simulink model "mancal_v2_corsi"  (R2013a)
settings: Solver=ode45  StartTime=0.0  StopTime=3  RelTol=1e-5
values from neighbouring files (symbols this model uses):
  dA = [1.435e2 3.335e-2]    [parametriza.m]    (also in parametrizaMancal.m)
  E = 3e9    (= 3000000000)    [parametriza.m]    (also in parametrizaMancal.m)
  gb = 0.4e-3    (= 0.0004)    [main.m]    (also in parametriza.m = 0.0003; parametrizaMancal.m)
  gi = 0.6e-3    (= 0.0006)    [main.m]    (also in parametriza.m = 0.0007; parametrizaMancal.m)
  Hb = 8e-3    (= 0.008)    [parametriza.m]    (also in parametrizaMancal.m)
  Kb = 46.53E3    (= 46530)    [main.m]    (also in parametriza.m = 58; parametrizaMancal.m = E*Hb*Ab/Lb)
  Ke = [3.8e-9 2.86e-3]    [parametrizaMancal.m]
  Km = 540e3    (= 540000)    [parametrizaMancal.m]
  L = [-57.6135 0.0908]    [main.m]    (also in parametriza.m = tf(Kb,[L2 R]); parametrizaMancal.m)
  Lb = 5.3e-3    (= 0.0053)    [parametriza.m]    (also in parametrizaMancal.m)
  m = 4.7e-5*7.86e3    (= 0.36942)    [main.m]    (also in parametriza.m = 0.375; parametrizaMancal.m)
  N = 300    [main.m]    (also in parametriza.m; parametrizaMancal.m)
  R = 4    [main.m]    (also in parametriza.m = 6.3; parametrizaMancal.m)
  Vmax = 30    [parametriza.m]    (also in parametrizaMancal.m)
undefined symbols (not defined in the file or in its folder): C
libraries: simulink x1, dspmathops x1
settings Model: SimulationMode=accelerator  Creator=leo  LastModifiedBy=rafa
settings DataIOCC: SignalLoggingSaveFormat=ModelDataLogs
settings OptimizationCC: AccelVerboseBuild=on
settings DebuggingCC: SolverPrmCheckMsg=none  MultiTaskDSMMsg=warning  MultiTaskCondExecSysMsg=none  StrictBusMsg=None
settings ModelReferenceCC: UpdateModelReferenceTargets=IfOutOfDate
settings SFSimCC: SFSimEcho=off
settings RTWCC: IncludeERTFirstTime=on

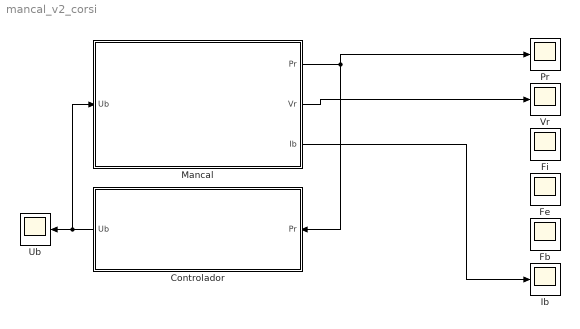
== system mancal_v2_corsi ==
  Controlador : Subsystem
  Fb : Scope
      settings: YMin=-200000  YMax=200000  SaveName=ScopeData6
  Fe : Scope
      settings: YMin=-500  YMax=25  SaveName=ScopeData2
  Fi : Scope
      settings: YMin=0  YMax=450  SaveName=ScopeData3
  Ib : Scope
      settings: YMin=-4  YMax=4  SaveName=ScopeData5
  Mancal : Subsystem
  Pr : Scope
      settings: TimeRange=3  YMin=-0.00045  YMax=0.00045
  Ub : Scope
      settings: TimeRange=0.1  YMin=0  YMax=10  SaveName=ScopeData10
  Vr : Scope
      settings: YMin=-45  YMax=45
  wires:
  Mancal/1(Pr) -> Pr/1, Controlador/1(Pr)
  Mancal/2(Vr) -> Vr/1
  ? -> Fe/1
  ? -> Fi/1
  Mancal/3(Ib) -> Ib/1
  ? -> Fb/1
  Controlador/1(Ub) -> Ub/1, Mancal/1(Ub)

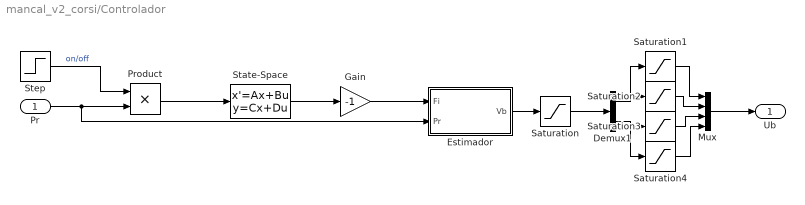
== system mancal_v2_corsi/Controlador ==
  Pr : Inport
  Demux1 : Demux  Outputs=2
  Estimador : Subsystem
  Gain : Gain  Gain=-1
  Mux : Mux
  Product : Product
  Saturation : Saturate  UpperLimit=Vmax  LowerLimit=-Vmax
  Saturation1 : Saturate  UpperLimit=Inf  LowerLimit=0
  Saturation2 : Saturate  UpperLimit=0  LowerLimit=-Inf
  Saturation3 : Saturate  UpperLimit=Inf  LowerLimit=0
  Saturation4 : Saturate  UpperLimit=0  LowerLimit=-Inf
  State-Space : StateSpace  A=ss([C 1; 1 C]).A  B=ss([C 1; 1 C]).B  C=ss([C 1; 1 C]).C  D=ss([C 1; 1 C]).D
  Step : Step  SampleTime=0
  Ub : Outport
  wires:
  Mux/1 -> Ub/1
  Saturation/1 -> Demux1/1
  Saturation4/1 -> Mux/4
  Saturation3/1 -> Mux/3
  Saturation2/1 -> Mux/2
  Saturation1/1 -> Mux/1
  Demux1/2 -> Saturation3/1, Saturation4/1
  Demux1/1 -> Saturation2/1, Saturation1/1
  Gain/1 -> Estimador/1(Fi)
  Estimador/1(Vb) -> Saturation/1
  State-Space/1 -> Gain/1
  Product/1 -> State-Space/1
  Pr/1 -> Product/2, Estimador/2(Pr)
  Step/1 -> Product/1  "on/off"

== system mancal_v2_corsi/Mancal ==
  Ub : Inport
  Batente : Subsystem
  Enrolamentos : Subsystem
  Imas : Subsystem
  Rotor : Subsystem
  Sum : Sum  Inputs=+++
  Pr : Outport
  Vr : Outport  Port=2
  Ib : Outport  Port=3
  wires:
  Sum/1 -> Rotor/1(Fr)  "F"
  Ub/1 -> Enrolamentos/1(Ub)
  Enrolamentos/1(Fe) -> Sum/3
  ? -> Ib/1
  Batente/1(Fb) -> Sum/1
  Rotor/1(Pr) -> Pr/1, Batente/1(Pr), Imas/1(Pr), Enrolamentos/2(Pr)
  Rotor/2(Vr) -> Batente/2(Vr), Vr/1
  Imas/1(Fi) -> Sum/2

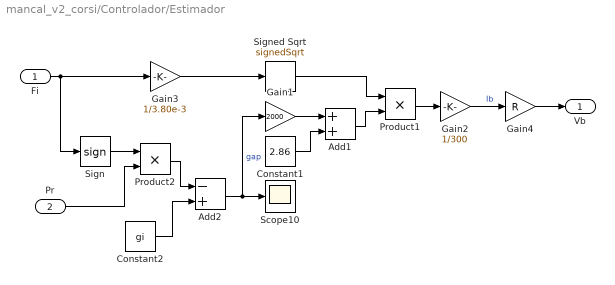
== system mancal_v2_corsi/Controlador/Estimador ==
  Fi : Inport
  Pr : Inport  Port=2
  Add1 : Sum
  Add2 : Sum  Inputs=-+
  Constant1 : Constant  Value=2.86
  Constant2 : Constant  Value=gi
  Gain1 : Gain  Gain=2000
  Gain2 : Gain  Gain=1/300
  Gain3 : Gain  Gain=1/3.80e-3
  Gain4 : Gain  Gain=R
  Product1 : Product
  Product2 : Product
  Scope10 : Scope
      settings: TimeRange=2.85171102661597  YMin=0.00015  YMax=0.0006  SaveName=ScopeData11
  Sign : Signum
  Signed Sqrt : Sqrt  Operator=signedSqrt  SaturateOnIntegerOverflow=on
  Vb : Outport
  wires:
  Constant2/1 -> Add2/2
  Product2/1 -> Add2/1
  Pr/1 -> Product2/2
  Sign/1 -> Product2/1
  Gain4/1 -> Vb/1
  Product1/1 -> Gain2/1
  Add2/1 -> Scope10/1, Gain1/1  "gap"
  Constant1/1 -> Add1/2
  Signed Sqrt/1 -> Product1/1
  Gain2/1 -> Gain4/1  "Ib"
  Gain3/1 -> Signed Sqrt/1
  Gain1/1 -> Add1/1
  Fi/1 -> Sign/1, Gain3/1
  Add1/1 -> Product1/2

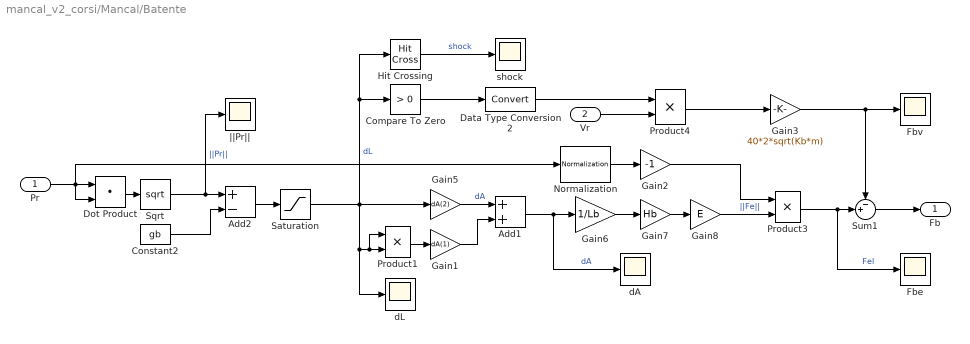
== system mancal_v2_corsi/Mancal/Batente ==
  Pr : Inport
  Vr : Inport  Port=2
  Add1 : Sum
  Add2 : Sum  Inputs=+-
  Compare To Zero : simulink/Logic and Bit Operations/Compare To Zero  relop=>  OutDataTypeStr=boolean
  Constant2 : Constant  Value=gb
  Data Type Conversion2 : DataTypeConversion
  Dot Product : DotProduct  InputSameDT=on  OutDataTypeStr=Inherit: Inherit via internal rule
  Fbe : Scope
      settings: TimeRange=0.0002829354553492485  YMin=-100000  YMax=100000  SaveName=ScopeData15
  Fbv : Scope
      settings: TimeRange=0.1  YMin=-225000  YMax=225000  SaveName=ScopeData8
  Gain1 : Gain  Gain=dA(1)
  Gain2 : Gain  Gain=-1
  Gain3 : Gain  Gain=40*2*sqrt(Kb*m)
  Gain5 : Gain  Gain=dA(2)
  Gain6 : Gain  Gain=1/Lb
  Gain7 : Gain  Gain=Hb
  Gain8 : Gain  Gain=E
  Hit Crossing : HitCross  HitCrossingDirection=rising
  Normalization : dspmathops/Normalization  NormType=2-norm  Bias=1e-10  NormOver=Each column  ColComp=on  Dimension=1  outputDataTypeStr=Inherit: Same as product output  outputLastDataTypeStr=Inherit: Same as product output  outputMin=[]  outputMax=[]  accumDataTypeStr=Inherit: Same as product output  accumLastDataTypeStr=Inherit: Same as product output  roundingMode=Floor  overflowMode=off
  Product1 : Product
  Product3 : Product
  Product4 : Product
  Saturation : Saturate  UpperLimit=Inf  LowerLimit=0
  Sqrt : Sqrt  SaturateOnIntegerOverflow=on
  Sum1 : Sum  Inputs=-+|
  dA : Scope
      settings: TimeRange=0.0002829354553492485  YMin=3.91545e-05  YMax=3.9158e-05  SaveName=ScopeData4
  dL : Scope
      settings: TimeRange=0.1  YMin=1.4215e-06  YMax=1.4315e-06  SaveName=ScopeData7
  shock : Scope
      settings: TimeRange=0.0002829354553492485  YMin=5.54637e-16  YMax=5.54639e-16  SaveName=ScopeData19
  ||Pr|| : Scope
      settings: TimeRange=0.0002829354553492485  YMin=-2.75  YMax=0  SaveName=ScopeData18
  Fb : Outport
  wires:
  Dot Product/1 -> Sqrt/1
  Gain8/1 -> Product3/2  "||Fe||"
  Compare To Zero/1 -> Data Type Conversion2/1
  Saturation/1 -> dL/1, Product1/1, Product1/2, Hit Crossing/1, Compare To Zero/1, Gain5/1  "dL"
  Add2/1 -> Saturation/1
  Sqrt/1 -> ||Pr||/1, Add2/1  "||Pr||"
  Constant2/1 -> Add2/2
  Gain6/1 -> Gain7/1
  Gain7/1 -> Gain8/1
  Product4/1 -> Gain3/1
  Product3/1 -> Sum1/2, Fbe/1  "Fel"
  Sum1/1 -> Fb/1
  Data Type Conversion2/1 -> Product4/1
  Product1/1 -> Gain1/1
  Gain5/1 -> Add1/1  "dA"
  Add1/1 -> dA/1, Gain6/1  "dA"
  Gain3/1 -> Fbv/1, Sum1/1
  Vr/1 -> Product4/2
  Normalization/1 -> Gain2/1
  Pr/1 -> Normalization/1, Dot Product/2, Dot Product/1
  Gain2/1 -> Product3/1
  Gain1/1 -> Add1/2
  Hit Crossing/1 -> shock/1  "shock"

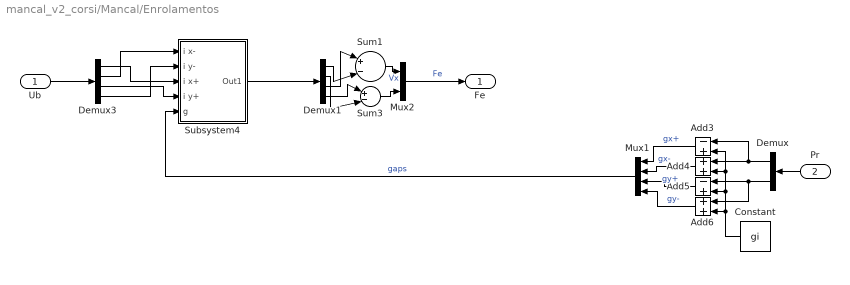
== system mancal_v2_corsi/Mancal/Enrolamentos ==
  Ub : Inport
  Pr : Inport  Port=2
  Add3 : Sum  Inputs=-+
  Add4 : Sum
  Add5 : Sum  Inputs=-+
  Add6 : Sum
  Constant : Constant  Value=gi
  Demux : Demux  Outputs=2
  Demux1 : Demux
  Demux3 : Demux
  Mux1 : Mux
  Mux2 : Mux  Inputs=2
  Subsystem4 : Subsystem
  Sum1 : Sum  Inputs=|+-|
  Sum3 : Sum  Inputs=|+-|
  Fe : Outport
  wires:
  Constant/1 -> Add5/2, Add4/2, Add3/2, Add6/2
  Mux2/1 -> Fe/1  "Fe"
  Sum3/1 -> Mux2/2
  Sum1/1 -> Mux2/1  "Vx"
  Add3/1 -> Mux1/1  "gx+"
  Add4/1 -> Mux1/2  "gx-"
  Add5/1 -> Mux1/3  "gy+"
  Add6/1 -> Mux1/4  "gy-"
  Demux/1 -> Add4/1, Add3/1
  Demux/2 -> Add5/1, Add6/1
  Pr/1 -> Demux/1
  Ub/1 -> Demux3/1
  Demux3/1 -> Subsystem4/3(i x+)
  Demux3/2 -> Subsystem4/1(i x-)
  Demux3/3 -> Subsystem4/4(i y+)
  Demux3/4 -> Subsystem4/2(i y-)
  Mux1/1 -> Subsystem4/5(g)  "gaps"
  Subsystem4/1(Out1) -> Demux1/1
  Demux1/3 -> Sum1/1
  Demux1/1 -> Sum1/2
  Demux1/4 -> Sum3/1
  Demux1/2 -> Sum3/2

== system mancal_v2_corsi/Mancal/Imas ==
  Pr : Inport
  Gain1 : Gain  Gain=Km
  Fi : Outport
  wires:
  Pr/1 -> Gain1/1
  Gain1/1 -> Fi/1  "Fm"

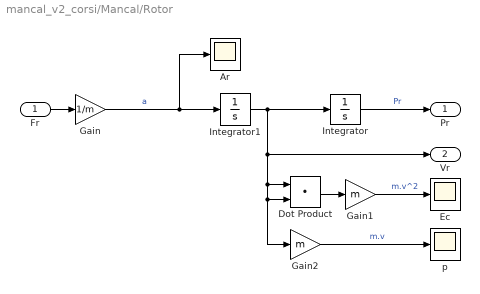
== system mancal_v2_corsi/Mancal/Rotor ==
  Fr : Inport
  Ar : Scope
      settings: TimeRange=1  YMin=-200000  YMax=200000  SaveName=ScopeData9
  Dot Product : DotProduct  InputSameDT=on  OutDataTypeStr=Inherit: Inherit via internal rule
  Ec : Scope
      settings: TimeRange=0.25  YMin=0  YMax=0.09  SaveName=ScopeData16
  Gain : Gain  Gain=1/m
  Gain1 : Gain  Gain=m
  Gain2 : Gain  Gain=m
  Integrator : Integrator  InitialCondition=[.001 .002]*1e-3  UpperSaturationLimit=Inf  LowerSaturationLimit=-Inf
  Integrator1 : Integrator
  p : Scope
      settings: TimeRange=1  YMin=-200000  YMax=200000  SaveName=ScopeData17
  Pr : Outport
  Vr : Outport  Port=2
  wires:
  Fr/1 -> Gain/1
  Integrator/1 -> Pr/1  "Pr"
  Gain/1 -> Ar/1, Integrator1/1  "a"
  Dot Product/1 -> Gain1/1
  Integrator1/1 -> Dot Product/1, Gain2/1, Dot Product/2, Vr/1, Integrator/1
  Gain2/1 -> p/1  "m.v"
  Gain1/1 -> Ec/1  "m.v^2"

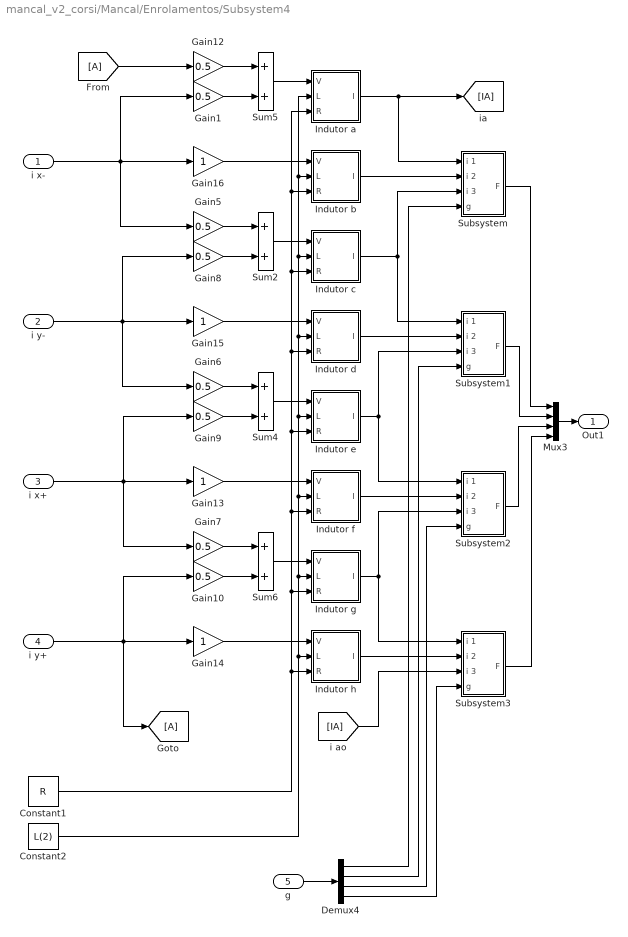
== system mancal_v2_corsi/Mancal/Enrolamentos/Subsystem4 ==
  i x- : Inport
  i y- : Inport  Port=2
  i x+ : Inport  Port=3
  i y+ : Inport  Port=4
  g : Inport  Port=5
  Constant1 : Constant  Value=R
  Constant2 : Constant  Value=L(2)
  Demux4 : Demux
  Gain{1,5..10,12} (8 alike) : Gain  Gain=0.5
  Gain{13..16} (4 alike) : Gain
  Indutor a : Subsystem
  Indutor b : Subsystem
  Indutor c : Subsystem
  Indutor d : Subsystem
  Indutor e : Subsystem
  Indutor f : Subsystem
  Indutor g : Subsystem
  Indutor h : Subsystem
  Mux3 : Mux
  Subsystem : Subsystem
  Subsystem1 : Subsystem
  Subsystem2 : Subsystem
  Subsystem3 : Subsystem
  Sum{2,4..6} (4 alike) : Sum
  Out1 : Outport
  wires:
  Sum6/1 -> Indutor g/1(V)
  i y+/1 -> [A], Gain10/1, Gain14/1
  [A] -> Gain12/1
  Gain13/1 -> Indutor f/1(V)
  Gain12/1 -> Sum5/1
  g/1 -> Demux4/1
  Demux4/3 -> Subsystem2/4(g)
  Indutor a/1(I) -> [IA], Subsystem/1(i 1)
  Subsystem/1(F) -> Mux3/1
  Demux4/1 -> Subsystem/4(g)
  Demux4/2 -> Subsystem1/4(g)
  Mux3/1 -> Out1/1
  Constant2/1 -> Indutor a/2(L), Indutor b/2(L), Indutor c/2(L), Indutor d/2(L), Indutor e/2(L), Indutor f/2(L), Indutor g/2(L), Indutor h/2(L)
  [IA] -> Subsystem3/3(i 3)
  Constant1/1 -> Indutor e/3(R), Indutor a/3(R), Indutor b/3(R), Indutor c/3(R), Indutor d/3(R), Indutor f/3(R), Indutor g/3(R), Indutor h/3(R)
  Demux4/4 -> Subsystem3/4(g)
  Subsystem3/1(F) -> Mux3/4
  Subsystem1/1(F) -> Mux3/2
  Indutor g/1(I) -> Subsystem2/3(i 3), Subsystem3/1(i 1)
  Indutor c/1(I) -> Subsystem/3(i 3), Subsystem1/1(i 1)
  Indutor d/1(I) -> Subsystem1/2(i 2)
  Indutor h/1(I) -> Subsystem3/2(i 2)
  Indutor e/1(I) -> Subsystem1/3(i 3), Subsystem2/1(i 1)
  Gain14/1 -> Indutor h/1(V)
  Gain15/1 -> Indutor d/1(V)
  Gain16/1 -> Indutor b/1(V)
  Indutor b/1(I) -> Subsystem/2(i 2)
  Sum5/1 -> Indutor a/1(V)
  Gain9/1 -> Sum4/2
  i x+/1 -> Gain7/1, Gain13/1, Gain9/1
  Gain10/1 -> Sum6/2
  Subsystem2/1(F) -> Mux3/3
  Indutor f/1(I) -> Subsystem2/2(i 2)
  i y-/1 -> Gain15/1, Gain8/1, Gain6/1
  Gain6/1 -> Sum4/1
  Sum4/1 -> Indutor e/1(V)
  Gain8/1 -> Sum2/2
  Gain7/1 -> Sum6/1
  Gain1/1 -> Sum5/2
  i x-/1 -> Gain1/1, Gain5/1, Gain16/1
  Sum2/1 -> Indutor c/1(V)
  Gain5/1 -> Sum2/1

== system mancal_v2_corsi/Mancal/Enrolamentos/Subsystem4/Indutor a ==
  V : Inport
  L : Inport  Port=2
  R : Inport  Port=3
  Divide2 : Product  Inputs=*/
  Integrator : Integrator
  Product : Product
  Sum1 : Sum  Inputs=|+-
  I : Outport
  wires:
  Divide2/1 -> Integrator/1
  Sum1/1 -> Divide2/1
  Integrator/1 -> Product/1, I/1
  Product/1 -> Sum1/2
  L/1 -> Divide2/2
  V/1 -> Sum1/1
  R/1 -> Product/2

== system mancal_v2_corsi/Mancal/Enrolamentos/Subsystem4/Indutor b ==
  V : Inport
  L : Inport  Port=2
  R : Inport  Port=3
  Divide2 : Product  Inputs=*/
  Integrator : Integrator
  Product : Product
  Sum1 : Sum  Inputs=|+-
  I : Outport
  wires:
  Divide2/1 -> Integrator/1
  Sum1/1 -> Divide2/1
  Integrator/1 -> Product/1, I/1
  Product/1 -> Sum1/2
  L/1 -> Divide2/2
  V/1 -> Sum1/1
  R/1 -> Product/2

== system mancal_v2_corsi/Mancal/Enrolamentos/Subsystem4/Indutor c ==
  V : Inport
  L : Inport  Port=2
  R : Inport  Port=3
  Divide2 : Product  Inputs=*/
  Integrator : Integrator
  Product : Product
  Sum1 : Sum  Inputs=|+-
  I : Outport
  wires:
  Divide2/1 -> Integrator/1
  Sum1/1 -> Divide2/1
  Integrator/1 -> Product/1, I/1
  Product/1 -> Sum1/2
  L/1 -> Divide2/2
  V/1 -> Sum1/1
  R/1 -> Product/2

== system mancal_v2_corsi/Mancal/Enrolamentos/Subsystem4/Indutor d ==
  V : Inport
  L : Inport  Port=2
  R : Inport  Port=3
  Divide2 : Product  Inputs=*/
  Integrator : Integrator
  Product : Product
  Sum1 : Sum  Inputs=|+-
  I : Outport
  wires:
  Divide2/1 -> Integrator/1
  Sum1/1 -> Divide2/1
  Integrator/1 -> Product/1, I/1
  Product/1 -> Sum1/2
  L/1 -> Divide2/2
  V/1 -> Sum1/1
  R/1 -> Product/2

== system mancal_v2_corsi/Mancal/Enrolamentos/Subsystem4/Indutor e ==
  V : Inport
  L : Inport  Port=2
  R : Inport  Port=3
  Divide2 : Product  Inputs=*/
  Integrator : Integrator
  Product : Product
  Sum1 : Sum  Inputs=|+-
  I : Outport
  wires:
  Divide2/1 -> Integrator/1
  Sum1/1 -> Divide2/1
  Integrator/1 -> Product/1, I/1
  Product/1 -> Sum1/2
  L/1 -> Divide2/2
  V/1 -> Sum1/1
  R/1 -> Product/2

== system mancal_v2_corsi/Mancal/Enrolamentos/Subsystem4/Indutor f ==
  V : Inport
  L : Inport  Port=2
  R : Inport  Port=3
  Divide2 : Product  Inputs=*/
  Integrator : Integrator
  Product : Product
  Sum1 : Sum  Inputs=|+-
  I : Outport
  wires:
  Divide2/1 -> Integrator/1
  Sum1/1 -> Divide2/1
  Integrator/1 -> Product/1, I/1
  Product/1 -> Sum1/2
  L/1 -> Divide2/2
  V/1 -> Sum1/1
  R/1 -> Product/2

== system mancal_v2_corsi/Mancal/Enrolamentos/Subsystem4/Indutor g ==
  V : Inport
  L : Inport  Port=2
  R : Inport  Port=3
  Divide2 : Product  Inputs=*/
  Integrator : Integrator
  Product : Product
  Sum1 : Sum  Inputs=|+-
  I : Outport
  wires:
  Divide2/1 -> Integrator/1
  Sum1/1 -> Divide2/1
  Integrator/1 -> Product/1, I/1
  Product/1 -> Sum1/2
  L/1 -> Divide2/2
  V/1 -> Sum1/1
  R/1 -> Product/2

== system mancal_v2_corsi/Mancal/Enrolamentos/Subsystem4/Indutor h ==
  V : Inport
  L : Inport  Port=2
  R : Inport  Port=3
  Divide2 : Product  Inputs=*/
  Integrator : Integrator
  Product : Product
  Sum1 : Sum  Inputs=|+-
  I : Outport
  wires:
  Divide2/1 -> Integrator/1
  Sum1/1 -> Divide2/1
  Integrator/1 -> Product/1, I/1
  Product/1 -> Sum1/2
  L/1 -> Divide2/2
  V/1 -> Sum1/1
  R/1 -> Product/2

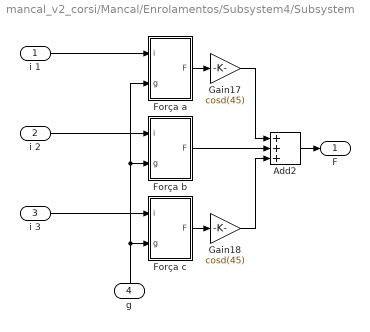
== system mancal_v2_corsi/Mancal/Enrolamentos/Subsystem4/Subsystem ==
  i 1 : Inport
  i 2 : Inport  Port=2
  i 3 : Inport  Port=3
  g : Inport  Port=4
  Add2 : Sum  Inputs=+++
  Força a : Subsystem
  Força b : Subsystem
  Força c : Subsystem
  Gain17 : Gain  Gain=cosd(45)
  Gain18 : Gain  Gain=cosd(45)
  F : Outport
  wires:
  Força a/1(F) -> Gain17/1
  g/1 -> Força c/2(g), Força b/2(g), Força a/2(g)
  Gain17/1 -> Add2/1
  Força c/1(F) -> Gain18/1
  Força b/1(F) -> Add2/2
  i 1/1 -> Força a/1(i)
  i 3/1 -> Força c/1(i)
  i 2/1 -> Força b/1(i)
  Gain18/1 -> Add2/3
  Add2/1 -> F/1

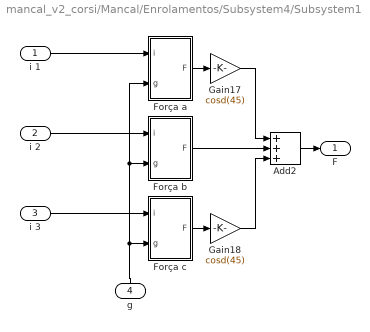
== system mancal_v2_corsi/Mancal/Enrolamentos/Subsystem4/Subsystem1 ==
  i 1 : Inport
  i 2 : Inport  Port=2
  i 3 : Inport  Port=3
  g : Inport  Port=4
  Add2 : Sum  Inputs=+++
  Força a : Subsystem
  Força b : Subsystem
  Força c : Subsystem
  Gain17 : Gain  Gain=cosd(45)
  Gain18 : Gain  Gain=cosd(45)
  F : Outport
  wires:
  Add2/1 -> F/1
  Gain18/1 -> Add2/3
  i 2/1 -> Força b/1(i)
  i 3/1 -> Força c/1(i)
  i 1/1 -> Força a/1(i)
  Força b/1(F) -> Add2/2
  Força c/1(F) -> Gain18/1
  Gain17/1 -> Add2/1
  g/1 -> Força a/2(g), Força b/2(g), Força c/2(g)
  Força a/1(F) -> Gain17/1

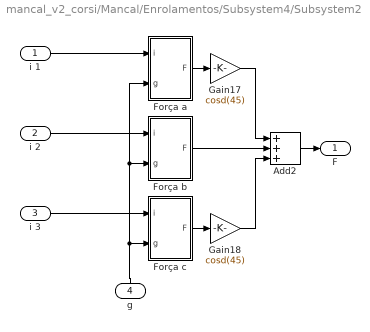
== system mancal_v2_corsi/Mancal/Enrolamentos/Subsystem4/Subsystem2 ==
  i 1 : Inport
  i 2 : Inport  Port=2
  i 3 : Inport  Port=3
  g : Inport  Port=4
  Add2 : Sum  Inputs=+++
  Força a : Subsystem
  Força b : Subsystem
  Força c : Subsystem
  Gain17 : Gain  Gain=cosd(45)
  Gain18 : Gain  Gain=cosd(45)
  F : Outport
  wires:
  Força a/1(F) -> Gain17/1
  g/1 -> Força c/2(g), Força b/2(g), Força a/2(g)
  Gain17/1 -> Add2/1
  Força c/1(F) -> Gain18/1
  Força b/1(F) -> Add2/2
  i 1/1 -> Força a/1(i)
  i 3/1 -> Força c/1(i)
  i 2/1 -> Força b/1(i)
  Gain18/1 -> Add2/3
  Add2/1 -> F/1

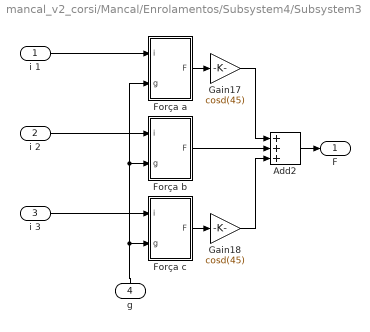
== system mancal_v2_corsi/Mancal/Enrolamentos/Subsystem4/Subsystem3 ==
  i 1 : Inport
  i 2 : Inport  Port=2
  i 3 : Inport  Port=3
  g : Inport  Port=4
  Add2 : Sum  Inputs=+++
  Força a : Subsystem
  Força b : Subsystem
  Força c : Subsystem
  Gain17 : Gain  Gain=cosd(45)
  Gain18 : Gain  Gain=cosd(45)
  F : Outport
  wires:
  Add2/1 -> F/1
  Gain18/1 -> Add2/3
  i 2/1 -> Força b/1(i)
  i 3/1 -> Força c/1(i)
  i 1/1 -> Força a/1(i)
  Força b/1(F) -> Add2/2
  Força c/1(F) -> Gain18/1
  Gain17/1 -> Add2/1
  g/1 -> Força a/2(g), Força b/2(g), Força c/2(g)
  Força a/1(F) -> Gain17/1

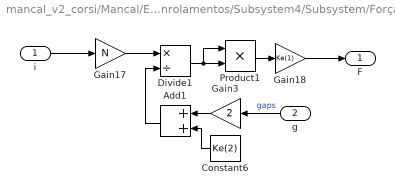
== system mancal_v2_corsi/Mancal/Enrolamentos/Subsystem4/Subsystem/Força a ==
  i : Inport
  g : Inport  Port=2
  Add1 : Sum
  Constant6 : Constant  Value=Ke(2)
  Divide1 : Product  Inputs=*/
  Gain17 : Gain  Gain=N
  Gain18 : Gain  Gain=Ke(1)
  Gain3 : Gain  Gain=2
  Product1 : Product
  F : Outport
  wires:
  Product1/1 -> Gain18/1
  Divide1/1 -> Product1/2, Product1/1
  Gain18/1 -> F/1
  i/1 -> Gain17/1
  Gain17/1 -> Divide1/1
  Gain3/1 -> Add1/1
  Constant6/1 -> Add1/2
  g/1 -> Gain3/1  "gaps"
  Add1/1 -> Divide1/2

== system mancal_v2_corsi/Mancal/Enrolamentos/Subsystem4/Subsystem/Força b ==
  i : Inport
  g : Inport  Port=2
  Add1 : Sum
  Constant6 : Constant  Value=Ke(2)
  Divide1 : Product  Inputs=*/
  Gain17 : Gain  Gain=N
  Gain18 : Gain  Gain=Ke(1)
  Gain3 : Gain  Gain=2
  Product1 : Product
  F : Outport
  wires:
  Product1/1 -> Gain18/1
  Divide1/1 -> Product1/2, Product1/1
  Gain18/1 -> F/1
  i/1 -> Gain17/1
  Gain17/1 -> Divide1/1
  Gain3/1 -> Add1/1
  Constant6/1 -> Add1/2
  g/1 -> Gain3/1  "gaps"
  Add1/1 -> Divide1/2

== system mancal_v2_corsi/Mancal/Enrolamentos/Subsystem4/Subsystem/Força c ==
  i : Inport
  g : Inport  Port=2
  Add1 : Sum
  Constant6 : Constant  Value=Ke(2)
  Divide1 : Product  Inputs=*/
  Gain17 : Gain  Gain=N
  Gain18 : Gain  Gain=Ke(1)
  Gain3 : Gain  Gain=2
  Product1 : Product
  F : Outport
  wires:
  Product1/1 -> Gain18/1
  Divide1/1 -> Product1/2, Product1/1
  Gain18/1 -> F/1
  i/1 -> Gain17/1
  Gain17/1 -> Divide1/1
  Gain3/1 -> Add1/1
  Constant6/1 -> Add1/2
  g/1 -> Gain3/1  "gaps"
  Add1/1 -> Divide1/2

== system mancal_v2_corsi/Mancal/Enrolamentos/Subsystem4/Subsystem1/Força a ==
  i : Inport
  g : Inport  Port=2
  Add1 : Sum
  Constant6 : Constant  Value=Ke(2)
  Divide1 : Product  Inputs=*/
  Gain17 : Gain  Gain=N
  Gain18 : Gain  Gain=Ke(1)
  Gain3 : Gain  Gain=2
  Product1 : Product
  F : Outport
  wires:
  Add1/1 -> Divide1/2
  g/1 -> Gain3/1  "gaps"
  Constant6/1 -> Add1/2
  Gain3/1 -> Add1/1
  Gain17/1 -> Divide1/1
  i/1 -> Gain17/1
  Gain18/1 -> F/1
  Divide1/1 -> Product1/1, Product1/2
  Product1/1 -> Gain18/1

== system mancal_v2_corsi/Mancal/Enrolamentos/Subsystem4/Subsystem1/Força b ==
  i : Inport
  g : Inport  Port=2
  Add1 : Sum
  Constant6 : Constant  Value=Ke(2)
  Divide1 : Product  Inputs=*/
  Gain17 : Gain  Gain=N
  Gain18 : Gain  Gain=Ke(1)
  Gain3 : Gain  Gain=2
  Product1 : Product
  F : Outport
  wires:
  Add1/1 -> Divide1/2
  g/1 -> Gain3/1  "gaps"
  Constant6/1 -> Add1/2
  Gain3/1 -> Add1/1
  Gain17/1 -> Divide1/1
  i/1 -> Gain17/1
  Gain18/1 -> F/1
  Divide1/1 -> Product1/1, Product1/2
  Product1/1 -> Gain18/1

== system mancal_v2_corsi/Mancal/Enrolamentos/Subsystem4/Subsystem1/Força c ==
  i : Inport
  g : Inport  Port=2
  Add1 : Sum
  Constant6 : Constant  Value=Ke(2)
  Divide1 : Product  Inputs=*/
  Gain17 : Gain  Gain=N
  Gain18 : Gain  Gain=Ke(1)
  Gain3 : Gain  Gain=2
  Product1 : Product
  F : Outport
  wires:
  Add1/1 -> Divide1/2
  g/1 -> Gain3/1  "gaps"
  Constant6/1 -> Add1/2
  Gain3/1 -> Add1/1
  Gain17/1 -> Divide1/1
  i/1 -> Gain17/1
  Gain18/1 -> F/1
  Divide1/1 -> Product1/1, Product1/2
  Product1/1 -> Gain18/1

== system mancal_v2_corsi/Mancal/Enrolamentos/Subsystem4/Subsystem2/Força a ==
  i : Inport
  g : Inport  Port=2
  Add1 : Sum
  Constant6 : Constant  Value=Ke(2)
  Divide1 : Product  Inputs=*/
  Gain17 : Gain  Gain=N
  Gain18 : Gain  Gain=Ke(1)
  Gain3 : Gain  Gain=2
  Product1 : Product
  F : Outport
  wires:
  Product1/1 -> Gain18/1
  Divide1/1 -> Product1/2, Product1/1
  Gain18/1 -> F/1
  i/1 -> Gain17/1
  Gain17/1 -> Divide1/1
  Gain3/1 -> Add1/1
  Constant6/1 -> Add1/2
  g/1 -> Gain3/1  "gaps"
  Add1/1 -> Divide1/2

== system mancal_v2_corsi/Mancal/Enrolamentos/Subsystem4/Subsystem2/Força b ==
  i : Inport
  g : Inport  Port=2
  Add1 : Sum
  Constant6 : Constant  Value=Ke(2)
  Divide1 : Product  Inputs=*/
  Gain17 : Gain  Gain=N
  Gain18 : Gain  Gain=Ke(1)
  Gain3 : Gain  Gain=2
  Product1 : Product
  F : Outport
  wires:
  Product1/1 -> Gain18/1
  Divide1/1 -> Product1/2, Product1/1
  Gain18/1 -> F/1
  i/1 -> Gain17/1
  Gain17/1 -> Divide1/1
  Gain3/1 -> Add1/1
  Constant6/1 -> Add1/2
  g/1 -> Gain3/1  "gaps"
  Add1/1 -> Divide1/2

== system mancal_v2_corsi/Mancal/Enrolamentos/Subsystem4/Subsystem2/Força c ==
  i : Inport
  g : Inport  Port=2
  Add1 : Sum
  Constant6 : Constant  Value=Ke(2)
  Divide1 : Product  Inputs=*/
  Gain17 : Gain  Gain=N
  Gain18 : Gain  Gain=Ke(1)
  Gain3 : Gain  Gain=2
  Product1 : Product
  F : Outport
  wires:
  Product1/1 -> Gain18/1
  Divide1/1 -> Product1/2, Product1/1
  Gain18/1 -> F/1
  i/1 -> Gain17/1
  Gain17/1 -> Divide1/1
  Gain3/1 -> Add1/1
  Constant6/1 -> Add1/2
  g/1 -> Gain3/1  "gaps"
  Add1/1 -> Divide1/2

== system mancal_v2_corsi/Mancal/Enrolamentos/Subsystem4/Subsystem3/Força a ==
  i : Inport
  g : Inport  Port=2
  Add1 : Sum
  Constant6 : Constant  Value=Ke(2)
  Divide1 : Product  Inputs=*/
  Gain17 : Gain  Gain=N
  Gain18 : Gain  Gain=Ke(1)
  Gain3 : Gain  Gain=2
  Product1 : Product
  F : Outport
  wires:
  Add1/1 -> Divide1/2
  g/1 -> Gain3/1  "gaps"
  Constant6/1 -> Add1/2
  Gain3/1 -> Add1/1
  Gain17/1 -> Divide1/1
  i/1 -> Gain17/1
  Gain18/1 -> F/1
  Divide1/1 -> Product1/1, Product1/2
  Product1/1 -> Gain18/1

== system mancal_v2_corsi/Mancal/Enrolamentos/Subsystem4/Subsystem3/Força b ==
  i : Inport
  g : Inport  Port=2
  Add1 : Sum
  Constant6 : Constant  Value=Ke(2)
  Divide1 : Product  Inputs=*/
  Gain17 : Gain  Gain=N
  Gain18 : Gain  Gain=Ke(1)
  Gain3 : Gain  Gain=2
  Product1 : Product
  F : Outport
  wires:
  Add1/1 -> Divide1/2
  g/1 -> Gain3/1  "gaps"
  Constant6/1 -> Add1/2
  Gain3/1 -> Add1/1
  Gain17/1 -> Divide1/1
  i/1 -> Gain17/1
  Gain18/1 -> F/1
  Divide1/1 -> Product1/1, Product1/2
  Product1/1 -> Gain18/1

== system mancal_v2_corsi/Mancal/Enrolamentos/Subsystem4/Subsystem3/Força c ==
  i : Inport
  g : Inport  Port=2
  Add1 : Sum
  Constant6 : Constant  Value=Ke(2)
  Divide1 : Product  Inputs=*/
  Gain17 : Gain  Gain=N
  Gain18 : Gain  Gain=Ke(1)
  Gain3 : Gain  Gain=2
  Product1 : Product
  F : Outport
  wires:
  Add1/1 -> Divide1/2
  g/1 -> Gain3/1  "gaps"
  Constant6/1 -> Add1/2
  Gain3/1 -> Add1/1
  Gain17/1 -> Divide1/1
  i/1 -> Gain17/1
  Gain18/1 -> F/1
  Divide1/1 -> Product1/1, Product1/2
  Product1/1 -> Gain18/1
